simulink model "plant_block"  (R2025a)
settings: Solver=ode1  StartTime=0.0  StopTime=300  RelTol=1e-3  EnableMultiTasking=on
settings Model: SimulationMode=external  Creator=Dro  LastModifiedBy=Matthew
settings SolverCC: AlgebraicLoopSolver=TrustRegion
settings DataIOCC: LimitDataPoints=on  SaveFormat=Array  SignalLoggingSaveFormat=ModelDataLogs  ReturnWorkspaceOutputs=off  SignalLoggingName=sigsOut
settings OptimizationCC: ExpressionDepthLimit=2147483647.0  InitFltsAndDblsToZero=on
settings DebuggingCC: SaveWithParameterizedLinksMsg=none  UnderspecifiedInitializationDetection=Classic  MergeDetectMultiDrivingBlocksExec=none  SignalResolutionControl=TryResolveAllWithWarning  MultiTaskDSMMsg=warning  MultiTaskCondExecSysMsg=none  FcnCallInpInsideContextMsg=warning  UnconnectedInputMsg=warning  UnconnectedOutputMsg=warning  UnconnectedLineMsg=warning  StateNameClashWarn=warning  SFUnexpectedBacktrackingDiag=warning  SFNoUnconditionalDefaultTransitionDiag=warning  SFExecutionAtInitializationDiag=none  ArithmeticOperatorsInVariantConditions=warning
settings HardwareCC: ProdBitPerLong=64.0  ProdHWDeviceType=Intel->x86-64 (Linux 64)  TargetBitPerLong=64.0  TargetBitPerPointer=64.0  TargetIntDivRoundTo=Zero  TargetEndianess=LittleEndian  TargetWordSize=64.0  TargetHWDeviceType=Intel->x86-64
settings ModelReferenceCC: EnableRefExpFcnMdlSchedulingChecks=on  PropagateSignalLabelsOutOfModel=off
settings SFSimCC: SimUseLocalCustomCode=off  CustomCodeUndefinedFunction=UseInterfaceOnly
settings RTWCC: SystemTargetFile=sldrt.tlc  TemplateMakefile=sldrt.tmf  RTWUseLocalCustomCode=off  RTWCompilerOptimization=on  GPUComputeCapability=3.5  Description=Simulink Desktop Real-Time
settings CodeAppCC: MaxIdLength=95.0  StateflowObjectComments=on
settings SimulinkDesktopRealTimeCC: ExtModeTransport=0.0  ExtModeStaticAllocSize=1000000.0  TargetLibSuffix=_sldrt.a  TargetPreCompLibLocation=C:\Program Files\MATLAB\R2025a\toolbox\sldrt\lib\win64  TargetLangStandard=C89/C90 (ANSI)  MultiwordLength=2048.0  DynamicStringBufferSize=256.0  ModelReferenceCompliant=off  ParMdlRefBuildCompliant=on  CompOptLevelCompliant=off  PreserveMATLABNamespacesInGeneratedCode=on  SubcomponentCodeInterfacePackaging=Reusable function  SupportVariableSizeSignals=off
settings ConfigComp: CovMetricSettings=dw  CovSaveCumulativeToWorkspaceVar=on  CovSaveSingleToWorkspaceVar=on  CovExternalEMLEnable=off

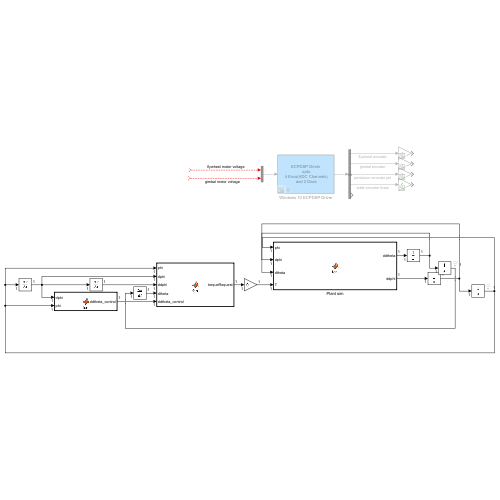
[thumbnail: Simulink's stored preview of the top-level diagram]
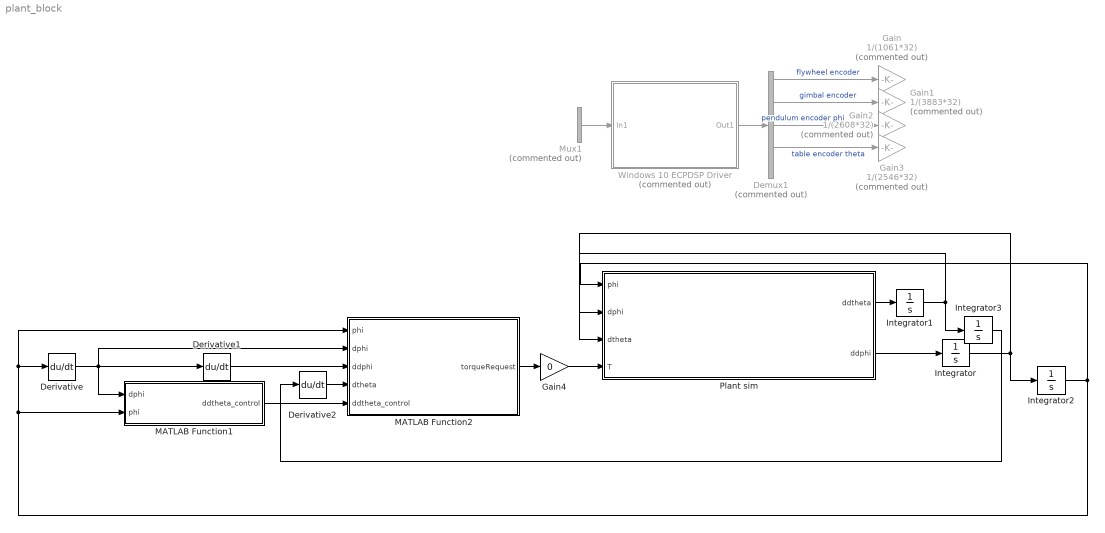
== system plant_block ==
  Demux1 : Demux  Commented=on  Outputs=5
      settings: DisplayOption=none
  Derivative : Derivative
  Derivative1 : Derivative
  Derivative2 : Derivative
  Gain : Gain  Commented=on  Gain=1/(1061*32)
  Gain1 : Gain  Commented=on  Gain=1/(3883*32)
  Gain2 : Gain  Commented=on  Gain=1/(2608*32)
  Gain3 : Gain  Commented=on  Gain=1/(2546*32)
  Gain4 : Gain  Gain=0
  Integrator : Integrator
  Integrator1 : Integrator
  Integrator2 : Integrator  InitialCondition=pi
  Integrator3 : Integrator
  MATLAB Function1 : MATLAB Function  TreatAsAtomicUnit=on
  MATLAB Function2 : MATLAB Function  TreatAsAtomicUnit=on
  Mux1 : Mux  Commented=on  Inputs=2
  Plant sim : MATLAB Function  TreatAsAtomicUnit=on
  Windows 10 ECPDSP Driver : Subsystem  Commented=on  mask{BaseAddr='0xD000', STime=0.008, TimeOutPer=500, HWAccess=on}
      mask prompts: BaseAddr "Base I/O Address"; STime "Sample Time (Sec)"; TimeOutPer "Timeout Period (500 ~ 2000)"; HWAccess "Hardware Access"
      mask Display: color('black');disp('ECPDSP Driver\n upto\n 4 Encs(ADC Channels)\n and 2 Dacs')
  wires:
  Mux1/1 -> Windows 10 ECPDSP Driver/1(In1)
  ? -> Mux1/1  "flywheel motor voltage"
  Demux1/1 -> Gain/1  "flywheel encoder"
  Demux1/2 -> Gain1/1  "gimbal encoder"
  Demux1/3 -> Gain2/1  "pendulum encoder phi"
  Demux1/4 -> Gain3/1  "table encoder theta"
  ? -> Mux1/2  "gimbal motor voltage"
  Windows 10 ECPDSP Driver/1(Out1) -> Demux1/1
  Plant sim/2(ddphi) -> Integrator/1
  Plant sim/1(ddtheta) -> Integrator1/1
  Integrator/1 -> Plant sim/2(dphi), Integrator2/1
  Integrator1/1 -> Integrator3/1, Plant sim/3(dtheta)
  Integrator2/1 -> Plant sim/1(phi), MATLAB Function2/1(phi), Derivative/1, MATLAB Function1/2(phi)
  Derivative/1 -> Derivative1/1, MATLAB Function2/2(dphi), MATLAB Function1/1(dphi)
  MATLAB Function1/1(ddtheta_control) -> MATLAB Function2/5(ddtheta_control)
  Derivative1/1 -> MATLAB Function2/3(ddphi)
  Derivative2/1 -> MATLAB Function2/4(dtheta)
  Integrator3/1 -> Derivative2/1
  MATLAB Function2/1(torqueRequest) -> Gain4/1
  Gain4/1 -> Plant sim/4(T)

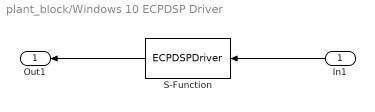
== system plant_block/Windows 10 ECPDSP Driver ==
  In1 : Inport
  S-Function : S-Function  FunctionName=ECPDSPDriver  Parameters=BaseAddr,STime,TimeOutPer,HWAccess  SFunctionDeploymentMode=off  EnableBusSupport=off
  Out1 : Outport
  wires:
  In1/1 -> S-Function/1
  S-Function/1 -> Out1/1

== matlab function plant_block/MATLAB Function1 ==
  data: dphi input; phi input; ddtheta_control output
function ddtheta_control = fcn(dphi, phi)
R = Rh
l = lcg;
r = 0; %reduced into J1_bar
M = 0; %reduced into J1_bar
g = grav;
c1 = 1; %friction of base
c2 = 0; %friction of pivot

J =  J1_bar% J - inertia of the table
Iyy = Jy 
I = Jz_bar%  I - inertia of the pendulum

k = 1
E = 0.5*I*dphi^2+m*g*l*(cos(phi)-1);
ddtheta_control = -k*E*dphi*cos(phi)/R;

== matlab function plant_block/Plant sim ==
  data: phi input; ddtheta output; dphi input; dtheta input; T input; ddphi output
function [ddtheta, ddphi] = fcn(phi, dphi, dtheta, T)

R = Rh
l = lcg;
r = 0; %reduced into J1_bar
M = 0; %reduced into J1_bar
g = grav;
c1 = 1; %friction of base
c2 = 0; %friction of pivot

J =  J1_bar% J - inertia of the table
Iyy = Jy 
I = Jz_bar%  I - inertia of the pendulum

ddtheta = -(R*m*sin(phi)*dphi^2*l + dtheta*m*sin(2*phi)*dphi*l^2 + Iyy*dtheta*sin(2*phi)*dphi - R*ddphi*m*cos(phi)*l - T + c1*dtheta)/(m*R^2 - m*l^2*cos(phi)^2 + m*l^2 - Iyy*cos(phi)^2 + Iyy + J);
ddphi = -(c2*dphi - 0.5000*Iyy*dtheta^2*sin(2*phi) + g*l*m*sin(phi) - 0.5000*dtheta^2*l^2*m*sin(2*phi) + (R*l*m*cos(phi)*(R*m*sin(phi)*dphi^2*l + dtheta*m*sin(2*phi)*dphi*l^2 + Iyy*dtheta*sin(2*phi)*dphi - T + c1*dtheta))/(m*R^2 - m*l^2*cos(phi)^2 + m*l^2 - Iyy*cos(phi)^2 + Iyy + J))/(I + l^2*m - (R^2*l^2*m^2*cos(phi)^2)/(m*R^2 - m*l^2*cos(phi)^2 + m*l^2 - Iyy*cos(phi)^2 + Iyy + J))
y = u;

== matlab function plant_block/MATLAB Function2 ==
  data: phi input; dphi input; ddphi input; dtheta input; torqueRequest output; ddtheta_control input
function torqueRequest = fcn(phi, dphi, ddphi,dtheta, ddtheta_control)
R = Rh;
l = lcg;
r = 0; %reduced into J1_bar
M = 0; %reduced into J1_bar
g = grav;
c1 = 1; %friction of base
c2 = 0; %friction of pivot

J =  J1_bar% J - inertia of the table
Iyy = Jy 
I = Jz_bar%  I - inertia of the pendulum

 torqueRequest = Iyy*ddtheta_control + J*ddtheta_control + c1*dtheta + ddtheta_control*m*R^2 + ddtheta_control*m*l^2 - Iyy*ddtheta_control*cos(phi)^2 + Iyy*dtheta*sin(2*phi)*dphi - ddtheta_control*m*l^2*cos(phi)^2 + m*sin(phi)*R*dphi^2*l + dtheta*m*sin(2*phi)*dphi*l^2 - ddphi*m*R*l*cos(phi)
